simulink model "OHC_NL_Boltzman_Function"  (R2019b)
settings: Solver=FixedStepAuto  StartTime=0.0  StopTime=testtime  RelTol=1e-3
InitFcn:
  | AN_InitFcn_Callback
StopFcn:
  | AN_StopFcn_Callback
undefined symbols (not defined in the file or in its folder): s0, s1, shift, x0, x1
settings Model: Creator=mblun  LastModifiedBy=cb50701
settings DataIOCC: SaveOutput=off  SaveTime=off
settings OptimizationCC: BlockReduction=off  ConditionallyExecuteInputs=off  DefaultParameterBehavior=Inlined
settings SFSimCC: CustomCodeUndefinedFunction=UseInterfaceOnly

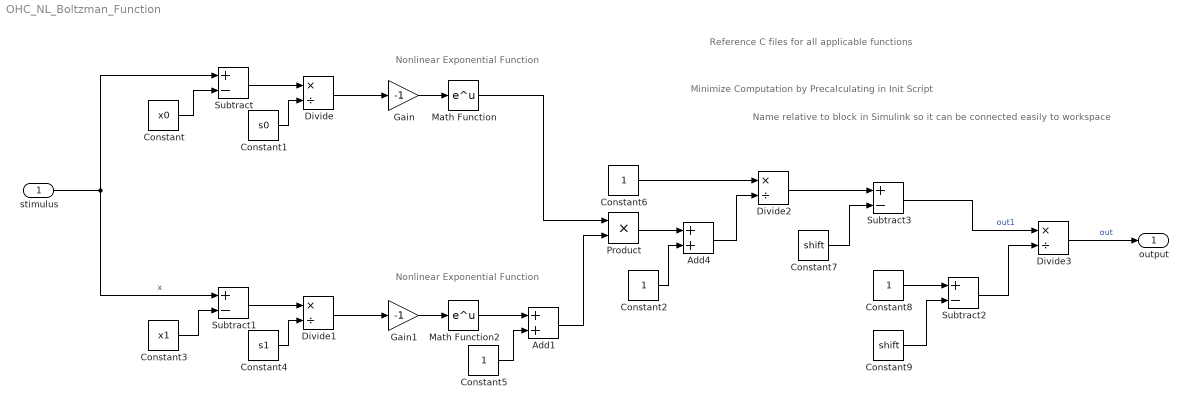
== system OHC_NL_Boltzman_Function ==
  note: Name relative to block in Simulink so it can be connected easily to workspace
  note: Minimize Computation by Precalculating in Init Script
  note: Reference C files for all applicable functions
  note: Nonlinear Exponential Function
  note: Nonlinear Exponential Function
  stimulus : Inport  OutDataTypeStr=double  PortDimensions=1  SampleTime=[2.0833333333333333e-05,0]
  Add1 : Sum
  Add4 : Sum
  Constant : Constant  Value=x0  SampleTime=-1
  Constant1 : Constant  Value=s0  SampleTime=-1
  Constant{2,5..6,8} (4 alike) : Constant  SampleTime=-1
  Constant3 : Constant  Value=x1  SampleTime=-1
  Constant4 : Constant  Value=s1  SampleTime=-1
  Constant7 : Constant  Value=shift  SampleTime=-1
  Constant9 : Constant  Value=shift  SampleTime=-1
  Divide{,1..3} (4 alike) : Product  Inputs=*/  SaturateOnIntegerOverflow=on  RndMeth=Zero
  Gain : Gain  Gain=-1
  Gain1 : Gain  Gain=-1
  Math Function : Math  SaturateOnIntegerOverflow=on
  Math Function2 : Math  SaturateOnIntegerOverflow=on
  Product : Product
  Subtract{,1..3} (4 alike) : Sum  Inputs=+-
  output : Outport  OutDataTypeStr=double  PortDimensions=1  SampleTime=[2.0833333333333333e-05,0]  VectorParamsAs1DForOutWhenUnconnected=off
  wires:
  Constant/1 -> Subtract/2
  stimulus/1 -> Subtract/1, Subtract1/1  "x"
  Subtract/1 -> Divide/1
  Constant1/1 -> Divide/2
  Divide/1 -> Gain/1
  Gain/1 -> Math Function/1
  Constant3/1 -> Subtract1/2
  Subtract1/1 -> Divide1/1
  Constant4/1 -> Divide1/2
  Divide1/1 -> Gain1/1
  Gain1/1 -> Math Function2/1
  Math Function2/1 -> Add1/1
  Constant5/1 -> Add1/2
  Add1/1 -> Product/2
  Constant6/1 -> Divide2/1
  Divide2/1 -> Subtract3/1
  Constant7/1 -> Subtract3/2
  Subtract3/1 -> Divide3/1  "out1"
  Constant8/1 -> Subtract2/1
  Constant9/1 -> Subtract2/2
  Subtract2/1 -> Divide3/2
  Divide3/1 -> output/1  "out"
  Math Function/1 -> Product/1
  Product/1 -> Add4/1
  Constant2/1 -> Add4/2
  Add4/1 -> Divide2/2
